simulink model "submodule"  (Simulink 9.0)
settings: Solver=ode5  StartTime=0.0  StopTime=1  MaxStep=1e-4  RelTol=1e-3
libraries: powerlib x5, simulink x1
settings Model: Creator=lenovo  LastModifiedBy=lenovo
settings DataIOCC: SaveFormat=Dataset
settings OptimizationCC: LifeSpan=auto
settings DebuggingCC: UnderspecifiedInitializationDetection=Simplified  MergeDetectMultiDrivingBlocksExec=error  SFUnexpectedBacktrackingDiag=error  SFNoUnconditionalDefaultTransitionDiag=error  SFExecutionAtInitializationDiag=warning
settings HardwareCC: ProdBitPerPointer=64  ProdBitPerSizeT=64  ProdBitPerPtrDiffT=64  ProdLargestAtomicFloat=Float  ProdIntDivRoundTo=Zero  ProdEndianess=LittleEndian  ProdWordSize=64  ProdHWDeviceType=Intel->x86-64 (Windows64)
settings ModelReferenceCC: PropagateSignalLabelsOutOfModel=on
settings CodeAppCC: StateflowObjectComments=off
settings GRTTargetCC: TargetLangStandard=C99 (ISO)
settings ConfigComp: CovMetricSettings=dwe  CovHtmlReporting=off  CovSaveCumulativeToWorkspaceVar=off  CovSaveSingleToWorkspaceVar=off  CovExternalEMLEnable=on

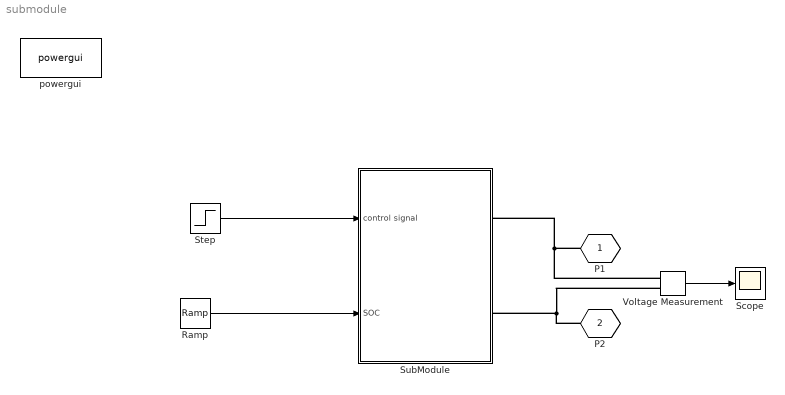
== system submodule ==
  Ramp : simulink/Sources/Ramp  slope=-1  start=0  X0=1
  Scope : Scope
  Step : Step  Time=0.5  Before=1  After=0  SampleTime=0
  SubModule : Subsystem
  Voltage Measurement : powerlib/Measurements/Voltage Measurement  PhasorSimulation=off  OutputType=Complex  PSBequivalent=0
  powergui : powerlib/powergui  Priority=1  SimulationMode=Discrete  SampleTime=50e-6  frequency=60  Iterations=50  frequencyindice=0  Pbase=100e6  ErrMax=1e-4  UnitsV=kV  UnitsW=MW  buscounter=0  FunctionMessages=off  echomessages=off  EnableUseOfTLC=off  CurrentSourceSwitches=off  DisableSnubberDevices=off  DisableRonSwitches=off  DisableVfSwitches=off  DisplayEquations=off  SolverType=Tustin/Backward Euler (TBE)  Interpol=off  ExternalGateDelay=off  methode=off  Ts=100  x0status=blocks  SPID=on  SwTol=0  HookPort=off  RestoreLinks=warning  ResistiveCurrentMeasurement=off  Frange=[0:2:500]  Ylog=off  Xlog=on  ShowGrid=off  save=off  variable=ZData  structure=0  ZoomFFT=off  StartTime=0.0  cycles=1  DisplayStyle=1  fundamental=60  FreqAxis=off  MaxFrequency=1000  frequencyindicesteady=1  RmsSteady=1  display=off
  P1 : PMIOPort  Tag=PMCPort  Port=1  Side=Right
  P2 : PMIOPort  Tag=PMCPort  Port=2  Side=Right
  wires:
  Step/1 -> SubModule/1(control signal)
  Ramp/1 -> SubModule/2(SOC)
  Voltage Measurement/1 -> Scope/1
  connections:
  P1/RConn1 -- Voltage Measurement/LConn1 -- SubModule/RConn1
  P2/RConn1 -- Voltage Measurement/LConn2 -- SubModule/RConn2

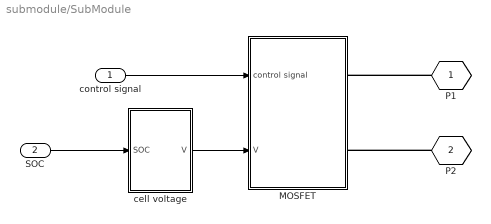
== system submodule/SubModule ==
  control signal : Inport
  SOC : Inport  Port=2
  MOSFET : Subsystem
  cell voltage : Subsystem
  P1 : PMIOPort  Tag=PMCPort  Port=1  Side=Right
  P2 : PMIOPort  Tag=PMCPort  Port=2  Side=Right
  wires:
  control signal/1 -> MOSFET/1(control signal)
  cell voltage/1(V) -> MOSFET/2(V)
  SOC/1 -> cell voltage/1(SOC)
  connections:
  P1/RConn1 -- MOSFET/RConn1
  P2/RConn1 -- MOSFET/RConn2

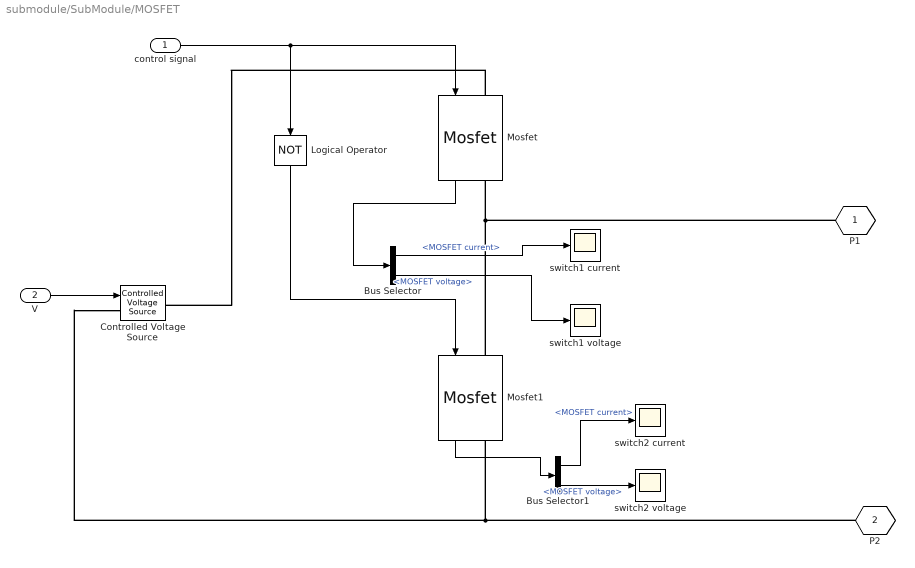
== system submodule/SubModule/MOSFET ==
  control signal : Inport
  V : Inport  Port=2
  Bus Selector : BusSelector  OutputSignals=MOSFET current,MOSFET voltage
  Bus Selector1 : BusSelector  OutputSignals=MOSFET current,MOSFET voltage
  Controlled Voltage Source : powerlib/Electrical Sources/Controlled Voltage Source  Initialize=on  Source_Type=AC  Amplitude=0  Phase=0  Frequency=0  Measurements=None
  Logical Operator : Logic  Operator=NOT  AllPortsSameDT=off  OutDataTypeStr=boolean
  Mosfet : powerlib/Power Electronics/Mosfet  Ron=0.0005  Lon=0  Rd=0.01  Vfd=0  IC=0  Rs=1e5  Cs=inf  Measurements=on
  Mosfet1 : powerlib/Power Electronics/Mosfet  Ron=0.0005  Lon=0  Rd=0.01  Vfd=0  IC=0  Rs=1e5  Cs=inf  Measurements=on
  switch1 current : Scope
  switch1 voltage : Scope
  switch2 current : Scope
  switch2 voltage : Scope
  P1 : PMIOPort  Tag=PMCPort  Port=1  Side=Right
  P2 : PMIOPort  Tag=PMCPort  Port=2  Side=Right
  wires:
  control signal/1 -> Logical Operator/1, Mosfet/1
  Mosfet/1 -> Bus Selector/1
  V/1 -> Controlled Voltage Source/1
  Bus Selector/1 -> switch1 current/1  "<MOSFET current>"
  Bus Selector/2 -> switch1 voltage/1  "<MOSFET voltage>"
  Bus Selector1/1 -> switch2 current/1  "<MOSFET current>"
  Bus Selector1/2 -> switch2 voltage/1  "<MOSFET voltage>"
  Logical Operator/1 -> Mosfet1/1
  Mosfet1/1 -> Bus Selector1/1
  connections:
  Mosfet1/RConn1 -- P2/RConn1 -- Controlled Voltage Source/LConn1
  Mosfet/RConn1 -- P1/RConn1 -- Mosfet1/LConn1
  Mosfet/LConn1 -- Controlled Voltage Source/RConn1

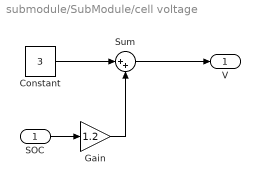
== system submodule/SubModule/cell voltage ==
  SOC : Inport
  Constant : Constant  Value=3
  Gain : Gain  Gain=1.2
  Sum : Sum  Inputs=|++
  V : Outport
  wires:
  Sum/1 -> V/1
  SOC/1 -> Gain/1
  Gain/1 -> Sum/2
  Constant/1 -> Sum/1
